simulink model "nonlinear_model_advanced_control_project (3)"  (R2020b)
settings: Solver=FixedStepAuto  StartTime=0.0  StopTime=10  FixedStep=0.01  RelTol=1e-3
values from neighbouring files (symbols this model uses):
  G = -J_RH*(M_M*L/2+M*l)*(J_RH+N^2*J_m+j)*g    (= -0.22537747671)    [HighWire_Artist_Dynamic_Model.m]    (also in llllllllllllllllllll.m = -0.0465293382657; lqr_advanced_project.m = -0.0465293382657; nnnnnnnn.m = -7422.6915)
  H = -N*K_m*J_RH    (= -0.00759948)    [HighWire_Artist_Dynamic_Model.m]    (also in llllllllllllllllllll.m = -0.00486576; lqr_advanced_project.m = -0.00486576; nnnnnnnn.m = -31.5)
  K_m = 0.0109    [HighWire_Artist_Dynamic_Model.m]    (also in llllllllllllllllllll.m; lqr_advanced_project.m; nnnnnnnn.m = 21)
  L_m = 0.145    [HighWire_Artist_Dynamic_Model.m]    (also in llllllllllllllllllll.m; lqr_advanced_project.m; nnnnnnnn.m = 0.5)
  N = 14    [HighWire_Artist_Dynamic_Model.m]    (also in llllllllllllllllllll.m = 3; lqr_advanced_project.m = 0; nnnnnnnn.m = 1)
  R_m = 1.6    [HighWire_Artist_Dynamic_Model.m]    (also in llllllllllllllllllll.m; lqr_advanced_project.m; nnnnnnnn.m = 40)
  T = (M_M*L/2+M*l)*(J_RH+N^2*J_m+j)*g    (= 4.52565214276)    [HighWire_Artist_Dynamic_Model.m]    (also in llllllllllllllllllll.m = 0.312697165764; lqr_advanced_project.m = 0.312697165764; nnnnnnnn.m = 4948.461)
  W = (J_M+M*l^2)*(J_RH+N^2*J_m+j)-(J_RH)^2    (= 0.0397505665657)    [HighWire_Artist_Dynamic_Model.m]    (also in llllllllllllllllllll.m = -0.0192235420783; lqr_advanced_project.m = -0.0192235420783; nnnnnnnn.m = 60.954)
  Z = (J_M+M*l^2)*(J_RH+N^2*J_m+j)^2-J_RH^2*(J_RH+N^2*J_m+j)    (= 0.251295170273)    [HighWire_Artist_Dynamic_Model.m]    (also in llllllllllllllllllll.m = -0.00839686182665; lqr_advanced_project.m = -0.00839686182665; nnnnnnnn.m = 418.75398)
settings Model: Creator=A family  LastModifiedBy=A family

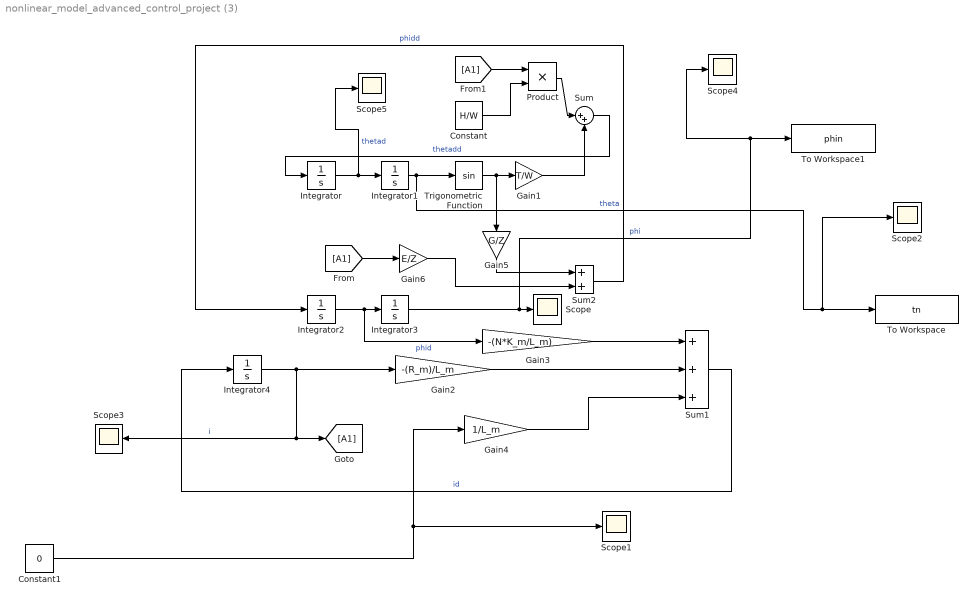
== system nonlinear_model_advanced_control_project (3) ==
  Constant : Constant  Value=H/W
  Constant1 : Constant  Value=0
  Gain1 : Gain  Gain=T/W
  Gain2 : Gain  Gain=-(R_m)/L_m
  Gain3 : Gain  Gain=-(N*K_m/L_m)
  Gain4 : Gain  Gain=1/L_m
  Gain5 : Gain  Gain=G/Z
  Gain6 : Gain  Gain=E/Z
  Integrator{,2..4} (4 alike) : Integrator
  Integrator1 : Integrator  InitialCondition=pi/180
  Product : Product
  Scope{,1..5} (6 alike) : Scope
  Sum : Sum  Inputs=|++
  Sum1 : Sum  Inputs=+++
  Sum2 : Sum
  To Workspace : ToWorkspace  VariableName=tn  SampleTime=-1
  To Workspace1 : ToWorkspace  VariableName=phin  SampleTime=-1
  Trigonometric Function : Trigonometry
  wires:
  Constant1/1 -> Scope1/1, Gain4/1
  Sum/1 -> Integrator/1  "thetadd"
  [A1] -> Gain6/1
  Sum1/1 -> Integrator4/1  "id"
  Gain3/1 -> Sum1/1
  Gain5/1 -> Sum2/1
  Sum2/1 -> Integrator2/1  "phidd"
  Integrator3/1 -> To Workspace1/1, Scope4/1, Scope/1  "phi"
  Trigonometric Function/1 -> Gain5/1, Gain1/1
  [A1] -> Product/1
  Gain6/1 -> Sum2/2
  Gain2/1 -> Sum1/2
  Integrator/1 -> Scope5/1, Integrator1/1  "thetad"
  Constant/1 -> Product/2
  Gain1/1 -> Sum/2
  Gain4/1 -> Sum1/3
  Integrator4/1 -> Scope3/1, [A1], Gain2/1  "i"
  Integrator2/1 -> Gain3/1, Integrator3/1  "phid"
  Integrator1/1 -> Scope2/1, To Workspace/1, Trigonometric Function/1  "theta"
  Product/1 -> Sum/1
